simulink model "t4"  (R2016a)
settings: Solver=VariableStepAuto  StartTime=0.0  StopTime=10.0  RelTol=1e-3
settings Model: Creator=admin  LastModifiedBy=admin

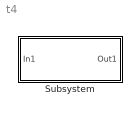
== system t4 ==
  Subsystem : Subsystem

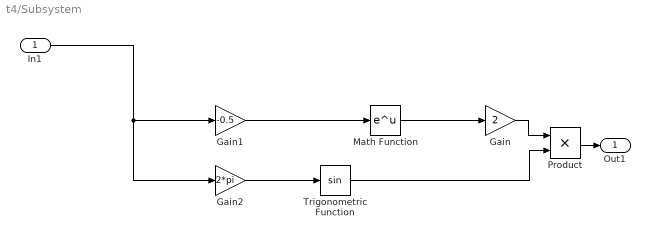
== system t4/Subsystem ==
  In1 : Inport
  Gain : Gain  Gain=2
  Gain1 : Gain  Gain=-0.5
  Gain2 : Gain  Gain=2*pi
  Math Function : Math  SaturateOnIntegerOverflow=on
  Product : Product
  Trigonometric Function : Trigonometry
  Out1 : Outport
  wires:
  Gain1/1 -> Math Function/1
  Math Function/1 -> Gain/1
  Gain2/1 -> Trigonometric Function/1
  Gain/1 -> Product/1
  Trigonometric Function/1 -> Product/2
  In1/1 -> Gain2/1, Gain1/1
  Product/1 -> Out1/1
